simulink model "traffic_moore_stateflow"  (R2020b)
settings: Solver=FixedStepDiscrete  StartTime=0.0  StopTime=inf  RelTol=1e-3  EnableMultiTasking=on
settings Model: EnablePacing=on  PacingRate=2  Creator=ADMIN  LastModifiedBy=ADMIN

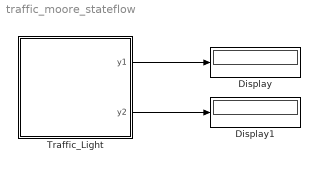
== system traffic_moore_stateflow ==
  Display : Display
  Display1 : Display
  Traffic_Light : Stateflow chart  TreatAsAtomicUnit=on
  wires:
  Traffic_Light/1(y1) -> Display/1
  Traffic_Light/2(y2) -> Display1/1

== stateflow chart traffic_moore_stateflow/Traffic_Light ==
  settings: stateMachineType=MOORE_MACHINE
  state Stop
    y1=RED;
    y2=GREEN;
  state StoptoTraffic
    y1=RED;
    y2=GREEN;
  state ReadytoMove
    y1=RED;
    y2=YELLOW
  state ReadytoStop
    y1=YELLOW;
    y2=RED;
  state Move
    y1=GREEN;
    y2=RED;
  (default) -> Stop
  Stop -> StoptoTraffic : after(5,sec)
  StoptoTraffic -> ReadytoMove : after(20,sec)
  ReadytoStop -> StoptoTraffic : after(5,sec)
  ReadytoMove -> Move : after(5,sec)
  Move -> ReadytoStop : after(20,sec)
  data: y1 output; y2 output; RED constant double =1; GREEN constant double =3; YELLOW constant double =2
